simulink model "p2_phase_loop_cosim"  (Simulink 6.4)
settings: Solver=FixedStepDiscrete  SolverMode=SingleTasking  StartTime=0.0  StopTime=5e-2  RelTol=1e-3
undefined symbols (not defined in the file or in its folder): pipeline_prec
libraries: modelsimlib x1
settings Model: LastModifiedBy=Administrador

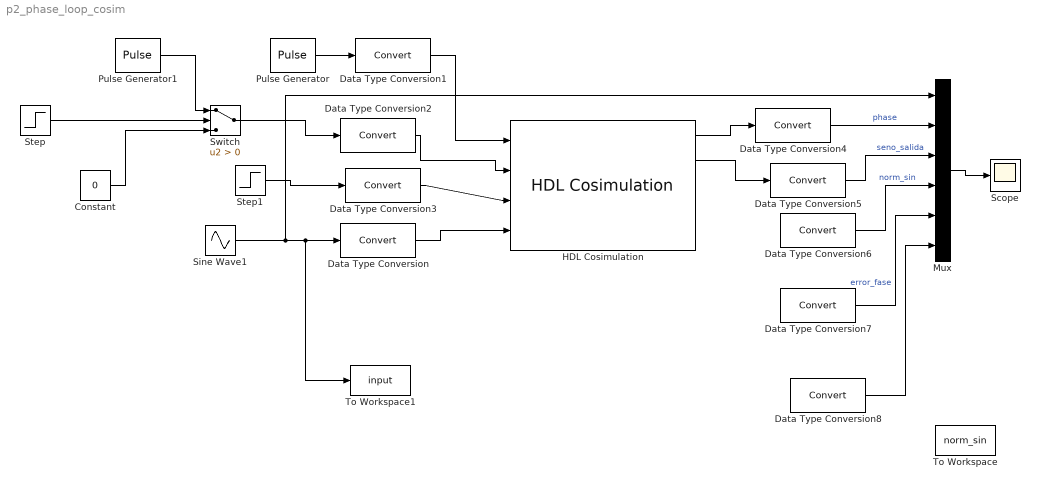
== system p2_phase_loop_cosim ==
  Constant : Constant  Value=0  OutDataType=sfix(16)  ConRadixGroup=Use specified scaling  OutScaling=2^0  SampleTime=1e-7  FramePeriod=inf
  Data Type Conversion : DataTypeConversion  OutDataTypeMode=Specify via dialog  OutScaling=2^(-pipeline_prec)  RndMeth=Nearest  SaturateOnIntegerOverflow=on
  Data Type Conversion1 : DataTypeConversion  OutDataTypeMode=boolean  SampleTime=1e-7
  Data Type Conversion2 : DataTypeConversion  OutDataTypeMode=boolean
  Data Type Conversion3 : DataTypeConversion  OutDataTypeMode=boolean
  Data Type Conversion{4..8} (5 alike) : DataTypeConversion
  HDL Cosimulation : modelsimlib/HDL Cosimulation  DialogController=modelsimddg.CoSim  DialogControllerArgs=DataTag0  PortPaths=/p2_phase_loop/clk;/p2_phase_loop/run;/p2_phase_loop/rst;/p2_phase_loop/input;/p2_phase_loop/phase;/p2_phase_loop/norm_sin;/p2_phase_loop/done;/p2_phase_loop/phase_det_i/phase_error;/p2_phase_loop/iir_1st_ord/o  PortModes=[1 1 1 1 2 2 2 2 2 ]  PortTimes=[1,1,1,1,1e-5,1e-5,1e-5,1e-5,1e-5]  PortSigns=[-1 -1 -1 -1 1 1 -1 1 1 ]  PortFracLengths=[0,0,0,0,pipeline_prec,pipeline_prec,0,pipeline_prec,pipeline_prec]  CommLocal=on  CommSharedMemory=off  CommPortNumber=4449  CommShowInfo=on  ClockModes=[]  ClockTimes=[]  TclPreSimCommand="echo \"Running Simulink Cosimulation block.\""  TclPostSimCommand="echo \"done\""  TimingMode=s  TimingScaleFactor=1  idxCellArray={'UNUSED_VAR'}
  Mux : Mux  Inputs=6
  Pulse Generator : DiscretePulseGenerator  PulseType=Time based  Period=1/(1e6)  PulseWidth=50
  Pulse Generator1 : DiscretePulseGenerator  PulseType=Time based  Period=0.1e-3  PulseWidth=2
  Scope : Scope
      settings: YMin=-3.5  YMax=3.5  MaxDataPoints=500000
  Sine Wave1 : Sin  Frequency=2*pi*50.05  Phase=1  SampleTime=1e-7
  Step : Step  Time=4*(1/1e6)  SampleTime=1e-7
  Step1 : Step  Time=6*(1/1e6)  Before=1  After=0  SampleTime=1e-7
  Switch : Switch  Criteria=u2 > Threshold  RndMeth=Nearest  ZeroCross=off  SampleTime=1e-7
  To Workspace : ToWorkspace  VariableName=norm_sin  SampleTime=-1  SaveFormat=Structure With Time
      settings: MaxDataPoints=3000
  To Workspace1 : ToWorkspace  VariableName=input  SampleTime=-1  SaveFormat=Structure With Time
      settings: MaxDataPoints=200000
  wires:
  Data Type Conversion/1 -> HDL Cosimulation/4
  Sine Wave1/1 -> Mux/1, Data Type Conversion/1, To Workspace1/1
  Pulse Generator/1 -> Data Type Conversion1/1
  Data Type Conversion1/1 -> HDL Cosimulation/1
  Switch/1 -> Data Type Conversion2/1
  Data Type Conversion2/1 -> HDL Cosimulation/2
  Step1/1 -> Data Type Conversion3/1
  Data Type Conversion3/1 -> HDL Cosimulation/3
  Constant/1 -> Switch/3
  Step/1 -> Switch/2
  Pulse Generator1/1 -> Switch/1
  HDL Cosimulation/1 -> Data Type Conversion4/1
  Data Type Conversion4/1 -> Mux/2  "phase"
  Data Type Conversion5/1 -> Mux/3  "seno_salida"
  Data Type Conversion6/1 -> Mux/4  "norm_sin"
  Data Type Conversion7/1 -> Mux/5  "error_fase"
  HDL Cosimulation/2 -> Data Type Conversion5/1
  Data Type Conversion8/1 -> Mux/6
  Mux/1 -> Scope/1
